simulink model "zad_no_10"  (R2017b)
settings: Solver=VariableStepAuto  StartTime=0.0  StopTime=10.0  RelTol=1e-3
undefined symbols (not defined in the file): A3_11, A3_12, A3_21, A3_22, B3_1, B3_2, K, L, Tp
settings Model: Creator=micha  LastModifiedBy=micha

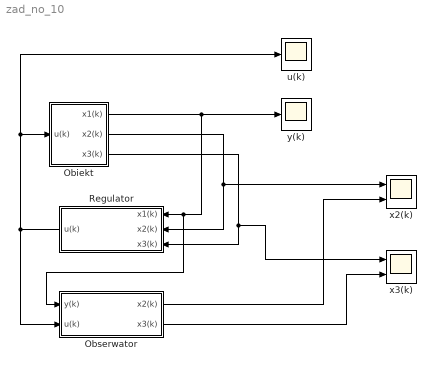
== system zad_no_10 ==
  Obiekt : Subsystem
  Obserwator : Subsystem
  Regulator : Subsystem
  u(k) : Scope
  x2(k) : Scope  NumInputPorts=2
  x3(k) : Scope  NumInputPorts=2
  y(k) : Scope
  wires:
  Obserwator/1(x2(k)) -> x2(k)/2
  Obiekt/3("x3(k) ") -> x3(k)/1, Regulator/3("x3(k) ")
  Regulator/1(u(k)) -> Obserwator/2(u(k)), Obiekt/1(u(k)), u(k)/1
  Obiekt/1(x1(k)) -> y(k)/1, Obserwator/1("y(k) "), Regulator/1("x1(k) ")
  Obiekt/2("x2(k) ") -> x2(k)/1, Regulator/2(x2(k))
  Obserwator/2("x3(k) ") -> x3(k)/2

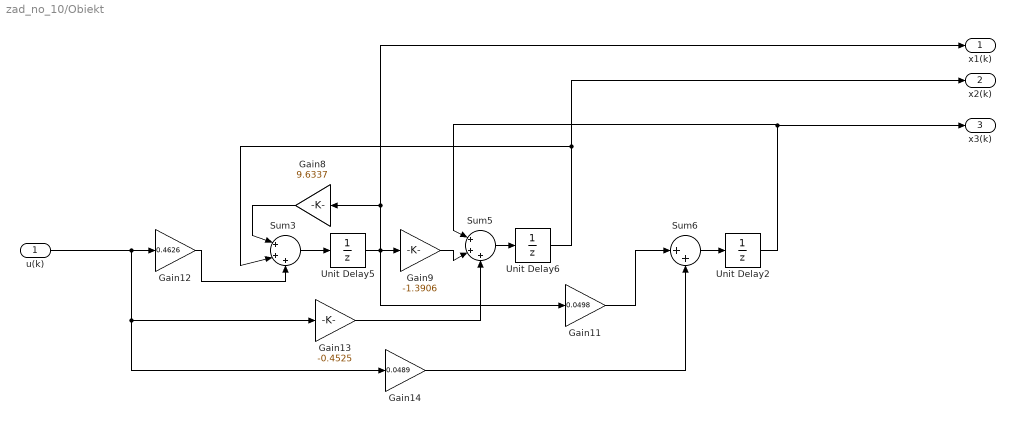
== system zad_no_10/Obiekt ==
  u(k) : Inport
  Gain11 : Gain  Gain=0.0498  ParamDataTypeStr=double
  Gain12 : Gain  Gain=0.4626  ParamDataTypeStr=double
  Gain13 : Gain  Gain=-0.4525  ParamDataTypeStr=double
  Gain14 : Gain  Gain=0.0489  ParamDataTypeStr=double
  Gain8 : Gain  Gain=9.6337  ParamDataTypeStr=double
  Gain9 : Gain  Gain=-1.3906  ParamDataTypeStr=double
  Sum3 : Sum  Inputs=|+++
  Sum5 : Sum  Inputs=|+++
  Sum6 : Sum  Inputs=|++
  Unit Delay2 : UnitDelay  InitialCondition=1  SampleTime=Tp
  Unit Delay5 : UnitDelay  InitialCondition=3  SampleTime=Tp
  Unit Delay6 : UnitDelay  InitialCondition=2  SampleTime=Tp
  x1(k) : Outport
  "x2(k) " : Outport  Port=2
  "x3(k) " : Outport  Port=3
  wires:
  Unit Delay6/1 -> "x2(k) "/1, Sum3/2
  Gain14/1 -> Sum6/2
  Unit Delay2/1 -> "x3(k) "/1, Sum5/1
  Unit Delay5/1 -> Gain11/1, x1(k)/1, Gain8/1, Gain9/1
  Gain13/1 -> Sum5/3
  Gain9/1 -> Sum5/2
  Gain12/1 -> Sum3/3
  Sum5/1 -> Unit Delay6/1
  Sum3/1 -> Unit Delay5/1
  Gain11/1 -> Sum6/1
  Gain8/1 -> Sum3/1
  Sum6/1 -> Unit Delay2/1
  u(k)/1 -> Gain12/1, Gain13/1, Gain14/1

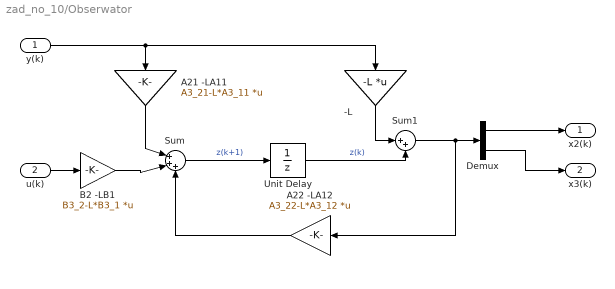
== system zad_no_10/Obserwator ==
  "y(k) " : Inport
  u(k) : Inport  Port=2
  -L : Gain  Gain=-L  Multiplication=Matrix(K*u)
  A21 -LA11 : Gain  Gain=A3_21-L*A3_11  Multiplication=Matrix(K*u)
  A22 -LA12 : Gain  Gain=A3_22-L*A3_12  Multiplication=Matrix(K*u)
  B2 -LB1 : Gain  Gain=B3_2-L*B3_1  Multiplication=Matrix(K*u)
  Demux : Demux  Outputs=2
  Sum : Sum  Inputs=|+++
  Sum1 : Sum  Inputs=|++
  Unit Delay : UnitDelay  SampleTime=Tp
  x2(k) : Outport
  "x3(k) " : Outport  Port=2
  wires:
  u(k)/1 -> B2 -LB1/1
  Demux/2 -> "x3(k) "/1
  Demux/1 -> x2(k)/1
  "y(k) "/1 -> A21 -LA11/1, -L/1
  B2 -LB1/1 -> Sum/2
  Sum/1 -> Unit Delay/1  "z(k+1)"
  -L/1 -> Sum1/1
  Unit Delay/1 -> Sum1/2  "z(k)"
  A22 -LA12/1 -> Sum/3
  A21 -LA11/1 -> Sum/1
  Sum1/1 -> Demux/1, A22 -LA12/1

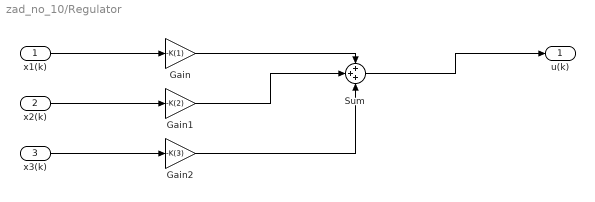
== system zad_no_10/Regulator ==
  "x1(k) " : Inport
  x2(k) : Inport  Port=2
  "x3(k) " : Inport  Port=3
  Gain : Gain  Gain=-K(1)
  Gain1 : Gain  Gain=-K(2)
  Gain2 : Gain  Gain=-K(3)
  Sum : Sum  Inputs=3
  u(k) : Outport
  wires:
  "x1(k) "/1 -> Gain/1
  x2(k)/1 -> Gain1/1
  "x3(k) "/1 -> Gain2/1
  Gain/1 -> Sum/1
  Gain1/1 -> Sum/2
  Gain2/1 -> Sum/3
  Sum/1 -> u(k)/1
